simulink model "Test_control_motores"  (R2023b)
settings: Solver=VariableStepAuto  StartTime=0.0  StopTime=10.0  RelTol=1e-3
settings Model: Creator=Felix  LastModifiedBy=Felix

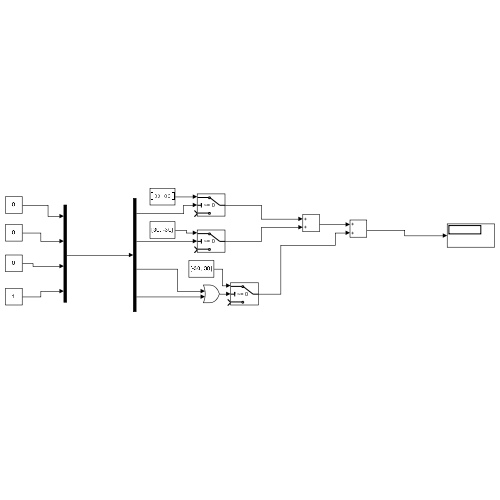
[thumbnail: Simulink's stored preview of the top-level diagram]
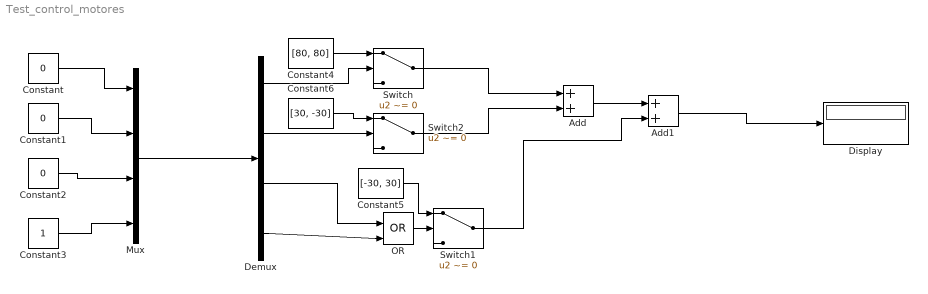
== system Test_control_motores ==
  Add : Sum
  Add1 : Sum
  Constant : Constant  Value=0
  Constant1 : Constant  Value=0
  Constant2 : Constant  Value=0
  Constant3 : Constant
  Constant4 : Constant  Value=[80, 80]  VectorParams1D=off
  Constant5 : Constant  Value=[-30, 30]  VectorParams1D=off
  Constant6 : Constant  Value=[30, -30]  VectorParams1D=off
  Demux : Demux
  Display : Display
  Mux : Mux
  OR : Logic  Operator=OR  IconShape=distinctive  AllPortsSameDT=off  OutDataTypeStr=boolean
  Switch : Switch  Criteria=u2 ~= 0  SaturateOnIntegerOverflow=off  InputSameDT=off
  Switch1 : Switch  Criteria=u2 ~= 0  SaturateOnIntegerOverflow=off  InputSameDT=off
  Switch2 : Switch  Criteria=u2 ~= 0  SaturateOnIntegerOverflow=off  InputSameDT=off
  wires:
  Switch2/1 -> Add/2
  Switch/1 -> Add/1
  Add1/1 -> Display/1
  Add/1 -> Add1/1
  Constant6/1 -> Switch2/1
  Constant2/1 -> Mux/3
  Constant3/1 -> Mux/4
  Switch1/1 -> Add1/2
  Demux/4 -> OR/2
  Constant1/1 -> Mux/2
  Mux/1 -> Demux/1
  Constant4/1 -> Switch/1
  Constant5/1 -> Switch1/1
  Demux/2 -> Switch2/2
  OR/1 -> Switch1/2
  Demux/3 -> OR/1
  Constant/1 -> Mux/1
  Demux/1 -> Switch/2
